simulink model "SimulationTest"  (R2023b)
settings: Solver=VariableStepAuto  StartTime=0.0  StopTime=10.0  RelTol=1e-3
settings Model: Creator=iceki  LastModifiedBy=iceki

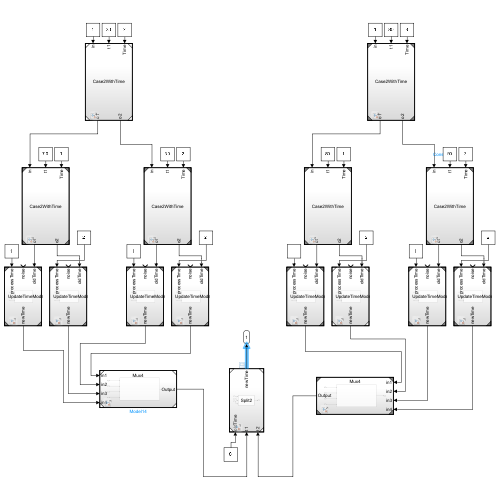
[thumbnail: Simulink's stored preview of the top-level diagram]
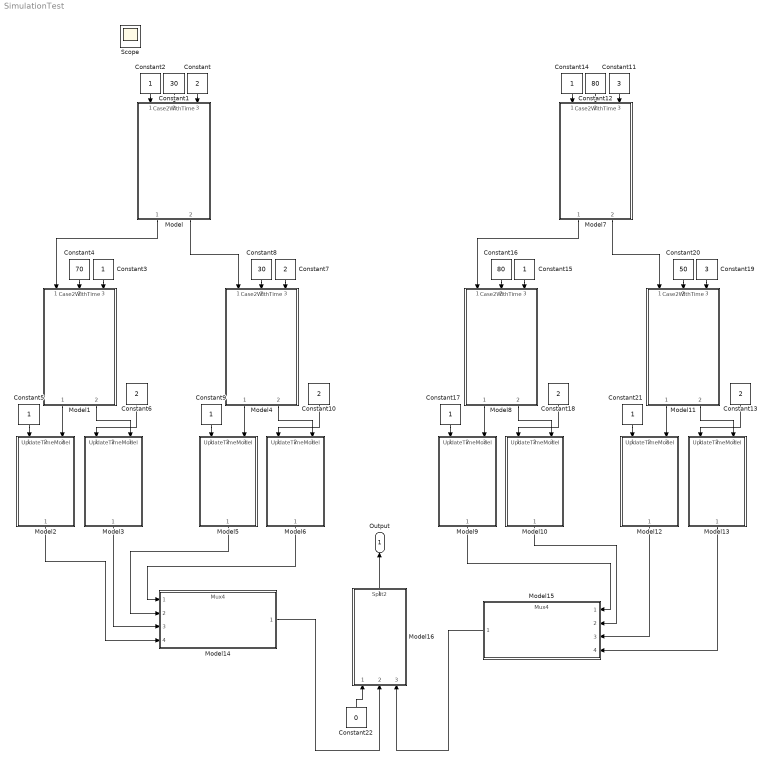
== system SimulationTest ==
  Constant{,6..7,10,13,18} (6 alike) : Constant  Value=2
  Constant1 : Constant  Value=30
  Constant11 : Constant  Value=3
  Constant12 : Constant  Value=80
  Constant{2..3,5,9,14..15,17,21} (8 alike) : Constant
  Constant16 : Constant  Value=80
  Constant19 : Constant  Value=3
  Constant20 : Constant  Value=50
  Constant22 : Constant  Value=0
  Constant4 : Constant  Value=70
  Constant8 : Constant  Value=30
  Model{,1,4,7..8,11} (6 alike) : ModelReference  ModelNameDialog=Case2WithTime.slx  SimulationMode=Normal  ModelReferenceVersion=1.10
  Model{2..3,5..6,9..10,12..13} (8 alike) : ModelReference  ModelNameDialog=UpdateTimeModel.slx  SimulationMode=Normal  ModelReferenceVersion=3.5
  Model14 : ModelReference  ModelNameDialog=Mux4.slx  SimulationMode=Normal  ModelReferenceVersion=1.5
  Model15 : ModelReference  ModelNameDialog=Mux4.slx  SimulationMode=Normal  ModelReferenceVersion=1.5
  Model16 : ModelReference  ModelNameDialog=Split2.slx  SimulationMode=Normal  ModelReferenceVersion=1.8
  Output : Outport
  Scope : Scope
  wires:
  Constant/1 -> Model/3
  Constant1/1 -> Model/2
  Constant2/1 -> Model/1
  Constant4/1 -> Model1/2
  Constant3/1 -> Model1/3
  Model/1 -> Model1/1
  Model1/1 -> Model2/3
  Constant5/1 -> Model2/1
  Model1/2 -> Model3/3
  Constant6/1 -> Model3/1
  Model4/1 -> Model5/3
  Model4/2 -> Model6/3
  Constant8/1 -> Model4/2
  Constant10/1 -> Model6/1
  Constant7/1 -> Model4/3
  Model/2 -> Model4/1
  Constant9/1 -> Model5/1
  Model8/1 -> Model9/3
  Model8/2 -> Model10/3
  Model7/2 -> Model11/1
  Model11/2 -> Model13/3
  Constant13/1 -> Model13/1
  Constant19/1 -> Model11/3
  Constant21/1 -> Model12/1
  Constant12/1 -> Model7/2
  Constant11/1 -> Model7/3
  Constant16/1 -> Model8/2
  Constant20/1 -> Model11/2
  Constant18/1 -> Model10/1
  Constant17/1 -> Model9/1
  Model11/1 -> Model12/3
  Constant14/1 -> Model7/1
  Model7/1 -> Model8/1
  Constant15/1 -> Model8/3
  Model6/1 -> Model14/1
  Model5/1 -> Model14/2
  Model3/1 -> Model14/3
  Model2/1 -> Model14/4
  Model9/1 -> Model15/1
  Model10/1 -> Model15/2
  Model12/1 -> Model15/3
  Model13/1 -> Model15/4
  Model14/1 -> Model16/2
  Model15/1 -> Model16/3
  Model16/1 -> Output/1
  Constant22/1 -> Model16/1
